simulink model "RT_ss2tf"  (R2013a)
settings: Solver=ode45  StartTime=0.0  StopTime=10.0  RelTol=1e-3
settings Model: Creator=mainster  LastModifiedBy=mainster

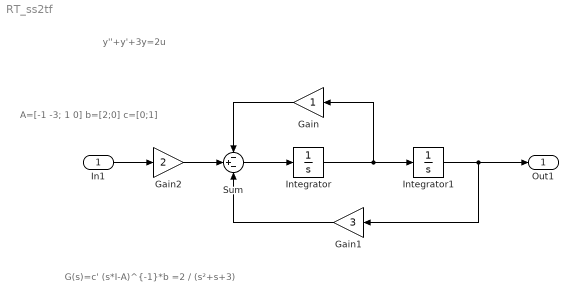
== system RT_ss2tf ==
  note: A=[-1 -3; 1 0]
      | b=[2;0]
      | c=[0;1]
  note: y''+y'+3y=2u
  note: G(s)=c' (s*I-A)^{-1}*b
      | =2 / (s²+s+3)
  In1 : Inport
  Gain : Gain
  Gain1 : Gain  Gain=3
  Gain2 : Gain  Gain=2
  Integrator : Integrator
  Integrator1 : Integrator
  Sum : Sum  Inputs=-+-
  Out1 : Outport
  wires:
  Gain/1 -> Sum/1
  Integrator/1 -> Integrator1/1, Gain/1
  Sum/1 -> Integrator/1
  Integrator1/1 -> Gain1/1, Out1/1
  Gain1/1 -> Sum/3
  Gain2/1 -> Sum/2
  In1/1 -> Gain2/1
